simulink model "chap7_2sim"  (Simulink 5.0)
settings: Solver=ode45  StartTime=0.0  StopTime=10  RelTol=1e-3
settings Model: LastModifiedBy=Administrator  ExtModeTrigMode=oneshot  ExtModeArmWhenConnect=off  LimitDataPoints=off  BooleanDataType=off

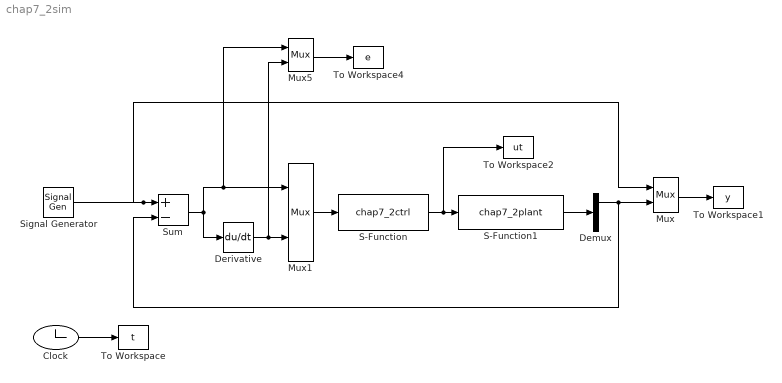
== system chap7_2sim ==
  Clock : Clock
  Demux : Demux  Outputs=2
  Derivative : Derivative
  Mux : Mux  Inputs=2
  Mux1 : Mux  Inputs=2
  Mux5 : Mux  Inputs=2
  S-Function : S-Function  FunctionName=chap7_2ctrl
  S-Function1 : S-Function  FunctionName=chap7_2plant
  Signal Generator : SignalGenerator
  Sum : Sum  Inputs=+-  SaturateOnIntegerOverflow=on  InputSameDT=on
  To Workspace : ToWorkspace  VariableName=t  SampleTime=-1  SaveFormat=Array
  To Workspace1 : ToWorkspace  VariableName=y  SampleTime=-1  SaveFormat=Array
  To Workspace2 : ToWorkspace  VariableName=ut  SampleTime=-1  SaveFormat=Array
  To Workspace4 : ToWorkspace  VariableName=e  SampleTime=-1  SaveFormat=Array
  wires:
  Clock/1 -> To Workspace/1
  S-Function1/1 -> Demux/1
  Demux/1 -> Mux/2, Sum/2
  Mux/1 -> To Workspace1/1
  Mux1/1 -> S-Function/1
  Derivative/1 -> Mux1/2, Mux5/2
  Sum/1 -> Derivative/1, Mux1/1, Mux5/1
  Signal Generator/1 -> Mux/1, Sum/1
  S-Function/1 -> S-Function1/1, To Workspace2/1
  Mux5/1 -> To Workspace4/1
